simulink model "PI_Controller_with_SupFuzzy"  (R2018b)
settings: Solver=ode23t  StartTime=0.0  StopTime=50  RelTol=1e-3
libraries: fuzblock x1
settings Model: Creator=admin  LastModifiedBy=admin

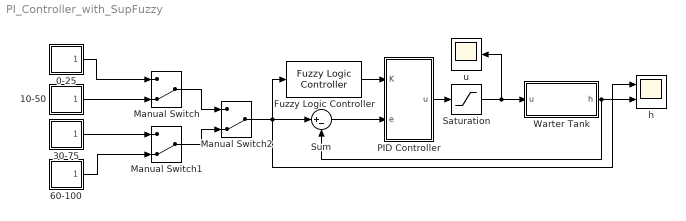
== system PI_Controller_with_SupFuzzy ==
  0-25 : Subsystem
  10-50 : Subsystem
  30-75 : Subsystem
  60-100 : Subsystem
  Fuzzy Logic Controller : fuzblock/Fuzzy Logic  Controller  FIS='FuzzySupWTank2.fis'  OutputSampleNumber=101  DataType=double  FuzzifiedInputs=off  RuleFiringStrengths=off  RuleOutputs=off  AggregatedOutputs=off  SimulateUsing=Interpreted execution  OutOfRangeInputValueMessage=warning  NoRuleFiredMessage=warning  EmptyOutputFuzzySetMessage=warning
  Manual Switch : ManualSwitch  CurrentSetting=0
  Manual Switch1 : ManualSwitch  CurrentSetting=0
  Manual Switch2 : ManualSwitch  CurrentSetting=0
  PID Controller : Subsystem
  Saturation : Saturate  UpperLimit=36  LowerLimit=0
  Sum : Sum  Inputs=|+-
  Warter Tank : Subsystem  mask{h0=0, Ah=100, k=300, Cd=0.6, a=1, g=981}
      mask prompts: h0 "Do cao ban dau (cm)"; Ah "Tiet dien ngang bon chua (cm2)"; k "He so ty le cong suat may bom"; Cd "He so xa"; a "Tiet dien van xa"; g "Gia toc trong truong"
  h : Scope  NumInputPorts=2
  u : Scope
  wires:
  Fuzzy Logic Controller/1 -> PID Controller/1(K)
  PID Controller/1(u) -> Saturation/1
  Saturation/1 -> u/1, Warter Tank/1(u)
  Manual Switch2/1 -> Fuzzy Logic Controller/1, h/1, Sum/1
  Warter Tank/1(h) -> Sum/2, h/2
  Sum/1 -> PID Controller/2(e)
  30-75/1(Out1) -> Manual Switch1/1
  10-50/1(Out1) -> Manual Switch/2
  0-25/1(Out1) -> Manual Switch/1
  Manual Switch1/1 -> Manual Switch2/2
  60-100/1(Out1) -> Manual Switch1/2
  Manual Switch/1 -> Manual Switch2/1

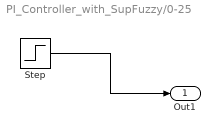
== system PI_Controller_with_SupFuzzy/0-25 ==
  Step : Step  Time=3  After=25  SampleTime=0
  Out1 : Outport
  wires:
  Step/1 -> Out1/1

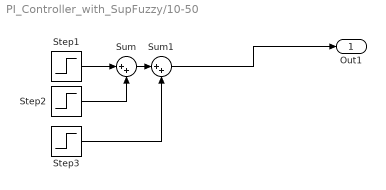
== system PI_Controller_with_SupFuzzy/10-50 ==
  Step1 : Step  Time=3  After=10  SampleTime=0
  Step2 : Step  Time=6  After=20  SampleTime=0
  Step3 : Step  Time=9  After=20  SampleTime=0
  Sum : Sum  Inputs=|++
  Sum1 : Sum  Inputs=|++
  Out1 : Outport
  wires:
  Sum/1 -> Sum1/1
  Step1/1 -> Sum/1
  Sum1/1 -> Out1/1
  Step3/1 -> Sum1/2
  Step2/1 -> Sum/2

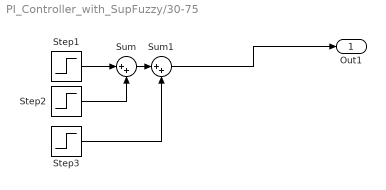
== system PI_Controller_with_SupFuzzy/30-75 ==
  Step1 : Step  Time=3  After=30  SampleTime=0
  Step2 : Step  Time=6  After=30  SampleTime=0
  Step3 : Step  Time=9  After=15  SampleTime=0
  Sum : Sum  Inputs=|++
  Sum1 : Sum  Inputs=|++
  Out1 : Outport
  wires:
  Sum/1 -> Sum1/1
  Step1/1 -> Sum/1
  Sum1/1 -> Out1/1
  Step3/1 -> Sum1/2
  Step2/1 -> Sum/2

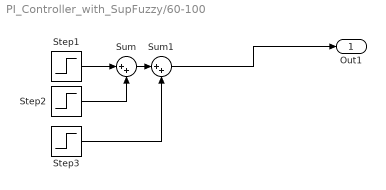
== system PI_Controller_with_SupFuzzy/60-100 ==
  Step1 : Step  Time=3  After=60  SampleTime=0
  Step2 : Step  Time=6  After=20  SampleTime=0
  Step3 : Step  Time=9  After=20  SampleTime=0
  Sum : Sum  Inputs=|++
  Sum1 : Sum  Inputs=|++
  Out1 : Outport
  wires:
  Sum/1 -> Sum1/1
  Step1/1 -> Sum/1
  Sum1/1 -> Out1/1
  Step3/1 -> Sum1/2
  Step2/1 -> Sum/2

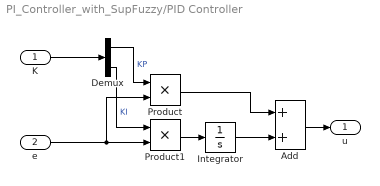
== system PI_Controller_with_SupFuzzy/PID Controller ==
  K : Inport
  e : Inport  Port=2
  Add : Sum
  Demux : Demux  Outputs=2
  Integrator : Integrator  UpperSaturationLimit=10  LowerSaturationLimit=-10
  Product : Product
  Product1 : Product
  u : Outport
  wires:
  Add/1 -> u/1
  K/1 -> Demux/1
  Demux/1 -> Product/1  "KP"
  e/1 -> Product/2, Product1/2
  Product/1 -> Add/1
  Demux/2 -> Product1/1  "KI"
  Product1/1 -> Integrator/1
  Integrator/1 -> Add/2

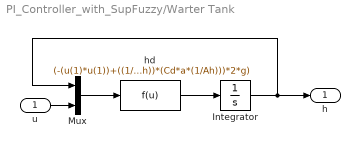
== system PI_Controller_with_SupFuzzy/Warter Tank ==
  u : Inport
  Integrator : Integrator  InitialCondition=h0  LimitOutput=on  UpperSaturationLimit=100  LowerSaturationLimit=0
  Mux : Mux  Inputs=2
  hd : Fcn  Expr=(-(u(1)*u(1))+((1/Ah)*k)*((1/Ah)*k)*u(2)*u(2))/(((Cd*a*(1/Ah))*(Cd*a*(1/Ah)))*2*g)
  h : Outport
  wires:
  hd/1 -> Integrator/1
  Integrator/1 -> Mux/1, h/1
  u/1 -> Mux/2
  Mux/1 -> hd/1
